simulink model "AnalysisSim"  (R2016a)
settings: Solver=VariableStepAuto  StartTime=0.0  StopTime=4.0  RelTol=1e-3
values from neighbouring files (symbols this model uses):
  C = Kphys    [DESIGN2_RobustFlutterSuppression-18-08-03.m]    (also in DESIGN2_RobustFlutterSuppression_18_08_03.m; Part1_Design_RobustFlutterSuppression.m; Part2_RobustnessAnalysis.m; ssctr.m = Ctmp)
  GeriFDsysPID2_IO = NdofwActSens(okeep,ikeep,AEC6,ModeShape,FEM,Vmps,aeroProp,massProp,     coeffdataPIDfull,actdata,sensdata)    [GenerateGeriModel.m]
  K = K*OutputBlend    [DESIGN1_RobustFlutterSuppression-18-07-27.m]    (also in DESIGN2_RobustFlutterSuppression-18-08-03.m; DESIGN2_RobustFlutterSuppression_18_08_03.m; Part1_Design_RobustFlutterSuppression.m)
  Vinf = VV    [DESIGN2_RobustFlutterSuppression-18-08-03.m]    (also in DESIGN2_RobustFlutterSuppression_18_08_03.m; Part1_Design_RobustFlutterSuppression.m; Part2_RobustnessAnalysis.m)
libraries: simulink_extras x4, dspsigattribs x4, cstblocks x1
settings Model: Creator=Julian  LastModifiedBy=Julian
settings GRTTargetCC: GeneratePreprocessorConditionals=Use local settings

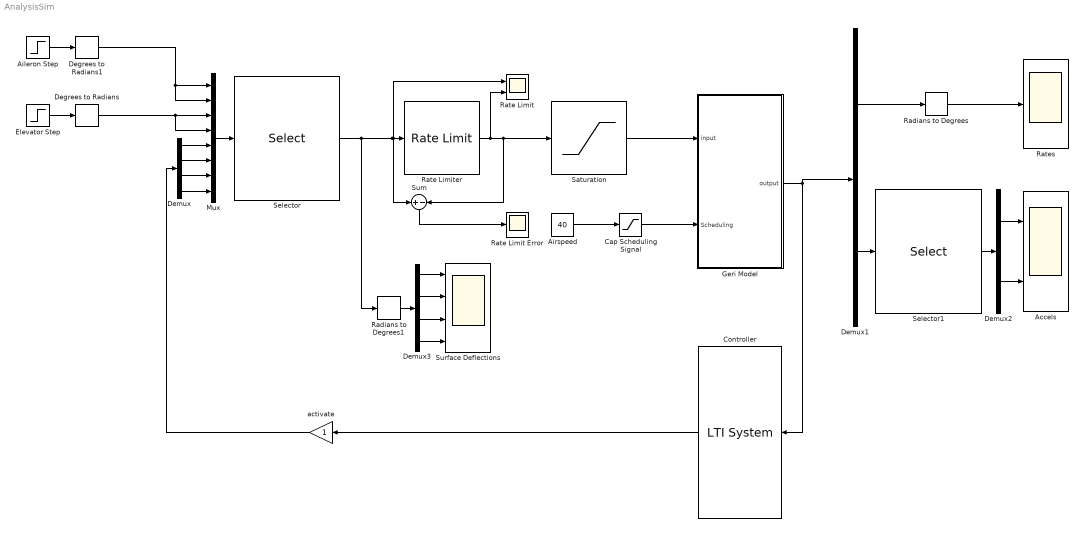
== system AnalysisSim ==
  Accels : Scope  NumInputPorts=2
  Aileron Step : Step  Time=3  After=0  SampleTime=0
  Airspeed : Constant  Value=40
  Cap Scheduling Signal : Saturate  UpperLimit=45  LowerLimit=25
  Controller : cstblocks/LTI System  sys=-C  IC=[]
  Degrees to Radians : simulink_extras/Transformations/Degrees to Radians
  Degrees to Radians1 : simulink_extras/Transformations/Degrees to Radians
  Demux : Demux
  Demux1 : Demux  Outputs=[2 6]
  Demux2 : Demux  Outputs=[3 3]
  Demux3 : Demux  Outputs=[2 2 2 2]
  Elevator Step : Step  SampleTime=0
  Geri Model : Subsystem
  Mux : Mux  Inputs=8
  Radians to Degrees : simulink_extras/Transformations/Radians to Degrees
  Radians to Degrees1 : simulink_extras/Transformations/Radians to Degrees
  Rate Limit : Scope  NumInputPorts=2
  Rate Limit Error : Scope
  Rate Limiter : RateLimiter  RisingSlewLimit=30/180*pi  FallingSlewLimit=-30/180*pi  SampleTimeMode=inherited
  Rates : Scope
  Saturation : Saturate  UpperLimit=30/180*pi  LowerLimit=-30/180*pi
  Selector : Selector  InputPortWidth=8  IndexOptions=Index vector (dialog)  Indices=[5 6 1 2 3 4 7 8]  OutputSizes=1
  Selector1 : Selector  InputPortWidth=6  IndexOptions=Index vector (dialog)  Indices=[6 2 5 4 1 3]  OutputSizes=1
  Sum : Sum  Inputs=+-
  Surface Deflections : Scope  NumInputPorts=4
  activate : Gain
  wires:
  Geri Model/1(output) -> Demux1/1, Controller/1
  Cap Scheduling Signal/1 -> Geri Model/2(Scheduling)
  Airspeed/1 -> Cap Scheduling Signal/1
  Mux/1 -> Selector/1
  Controller/1 -> activate/1
  Elevator Step/1 -> Degrees to Radians/1
  Demux/4 -> Mux/8
  Demux/3 -> Mux/7
  Demux/2 -> Mux/6
  Demux/1 -> Mux/5
  Degrees to Radians/1 -> Mux/4, Mux/3
  Aileron Step/1 -> Degrees to Radians1/1
  Degrees to Radians1/1 -> Mux/1, Mux/2
  Selector/1 -> Sum/1, Rate Limit/1, Rate Limiter/1, Radians to Degrees1/1
  Demux1/1 -> Radians to Degrees/1
  Demux1/2 -> Selector1/1
  Selector1/1 -> Demux2/1
  Demux2/1 -> Accels/1
  Demux2/2 -> Accels/2
  activate/1 -> Demux/1
  Radians to Degrees/1 -> Rates/1
  Radians to Degrees1/1 -> Demux3/1
  Demux3/1 -> Surface Deflections/1
  Demux3/3 -> Surface Deflections/3
  Demux3/2 -> Surface Deflections/2
  Demux3/4 -> Surface Deflections/4
  Saturation/1 -> Geri Model/1(input)
  Rate Limiter/1 -> Sum/2, Saturation/1, Rate Limit/2
  Sum/1 -> Rate Limit Error/1

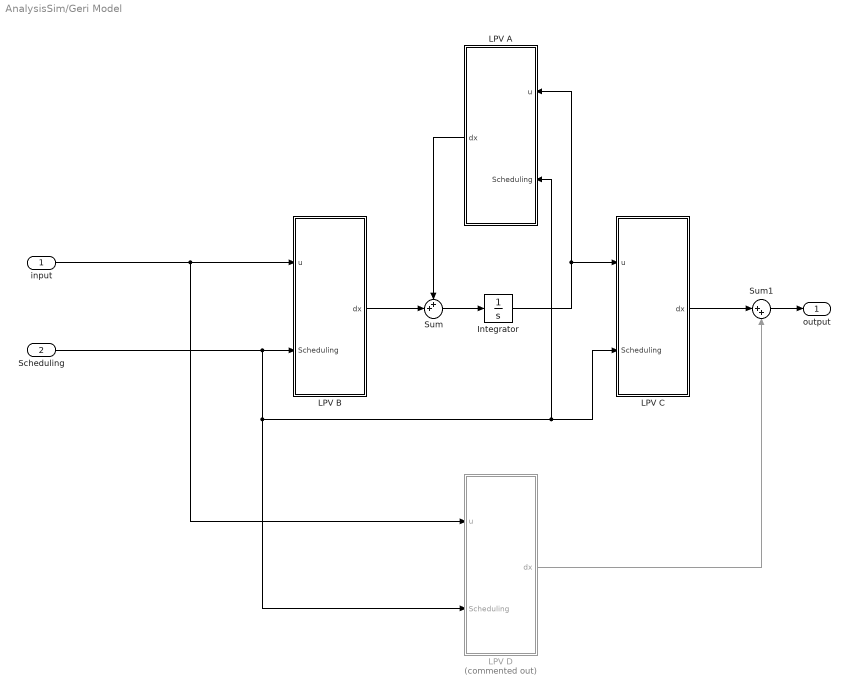
== system AnalysisSim/Geri Model ==
  input : Inport
  Scheduling : Inport  Port=2
  Integrator : Integrator  InitialCondition=zeros(size(GeriFDsysPID2_IO.a,1),1)
  LPV A : Subsystem
  LPV B : Subsystem
  LPV C : Subsystem
  LPV D : Subsystem  Commented=on
  Sum : Sum  Inputs=++|
  Sum1 : Sum  Inputs=|++
  output : Outport
  wires:
  LPV C/1(dx) -> Sum1/1
  Sum/1 -> Integrator/1
  Integrator/1 -> LPV C/1(u), LPV A/1(u)
  input/1 -> LPV D/1(u), LPV B/1(u)
  Scheduling/1 -> LPV B/2(Scheduling), LPV D/2(Scheduling), LPV C/2(Scheduling), LPV A/2(Scheduling)
  LPV B/1(dx) -> Sum/2
  LPV A/1(dx) -> Sum/1
  Sum1/1 -> output/1
  LPV D/1(dx) -> Sum1/2

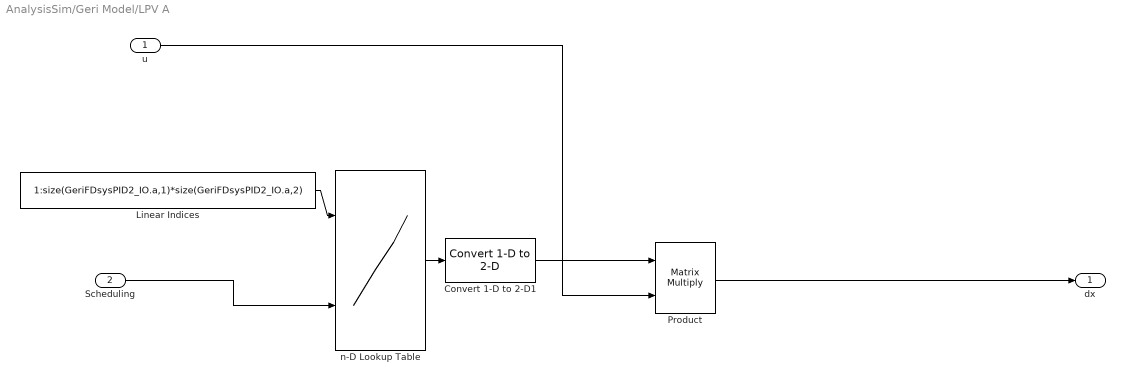
== system AnalysisSim/Geri Model/LPV A ==
  u : Inport
  Scheduling : Inport  Port=2
  Convert 1-D to 2-D1 : dspsigattribs/Convert 1-D to 2-D  M=size(GeriFDsysPID2_IO.a,1)  N=size(GeriFDsysPID2_IO.a,2)  frameBasedOut=off
  Linear Indices : Constant  Value=1:size(GeriFDsysPID2_IO.a,1)*size(GeriFDsysPID2_IO.a,2)
  Product : Product  Multiplication=Matrix(*)
  n-D Lookup Table : Lookup_n-D  BreakpointsForDimension1=1:size(GeriFDsysPID2_IO.a,1)*size(GeriFDsysPID2_IO.a,2)  BreakpointsForDimension2=Vinf  BreakpointsForDimension3=K.Parameter.q2.GridData  BreakpointsForDimension4=K.Parameter.q3.GridData  BreakpointsForDimension5=q3.GridData  BeginIndexSearchUsingPreviousIndexResult=on  Table=reshape(GeriFDsysPID2_IO.a,[size(GeriFDsysPID2_IO.a,1)*size(GeriFDsysPID2_IO.a,2), numel(Vinf)])  ExtrapMethod=Clip  UseLastTableValue=on  InternalRulePriority=Speed  RndMeth=Simplest  InputSameDT=on
  dx : Outport
  wires:
  Scheduling/1 -> n-D Lookup Table/2
  u/1 -> Product/2
  Linear Indices/1 -> n-D Lookup Table/1
  Convert 1-D to 2-D1/1 -> Product/1
  n-D Lookup Table/1 -> Convert 1-D to 2-D1/1
  Product/1 -> dx/1

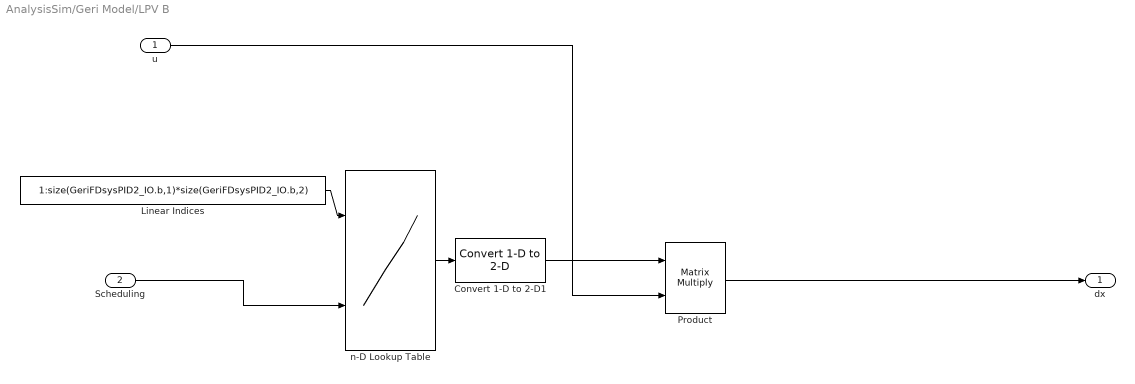
== system AnalysisSim/Geri Model/LPV B ==
  u : Inport
  Scheduling : Inport  Port=2
  Convert 1-D to 2-D1 : dspsigattribs/Convert 1-D to 2-D  M=size(GeriFDsysPID2_IO.b,1)  N=size(GeriFDsysPID2_IO.b,2)  frameBasedOut=off
  Linear Indices : Constant  Value=1:size(GeriFDsysPID2_IO.b,1)*size(GeriFDsysPID2_IO.b,2)
  Product : Product  Multiplication=Matrix(*)
  n-D Lookup Table : Lookup_n-D  BreakpointsForDimension1=1:size(GeriFDsysPID2_IO.b,1)*size(GeriFDsysPID2_IO.b,2)  BreakpointsForDimension2=Vinf  BreakpointsForDimension3=K.Parameter.q2.GridData  BreakpointsForDimension4=K.Parameter.q3.GridData  BreakpointsForDimension5=q3.GridData  BeginIndexSearchUsingPreviousIndexResult=on  Table=reshape(GeriFDsysPID2_IO.b,[size(GeriFDsysPID2_IO.b,1)*size(GeriFDsysPID2_IO.b,2), numel(Vinf)])  ExtrapMethod=Clip  UseLastTableValue=on  InternalRulePriority=Speed  RndMeth=Simplest  InputSameDT=on
  dx : Outport
  wires:
  Product/1 -> dx/1
  n-D Lookup Table/1 -> Convert 1-D to 2-D1/1
  Convert 1-D to 2-D1/1 -> Product/1
  Linear Indices/1 -> n-D Lookup Table/1
  u/1 -> Product/2
  Scheduling/1 -> n-D Lookup Table/2

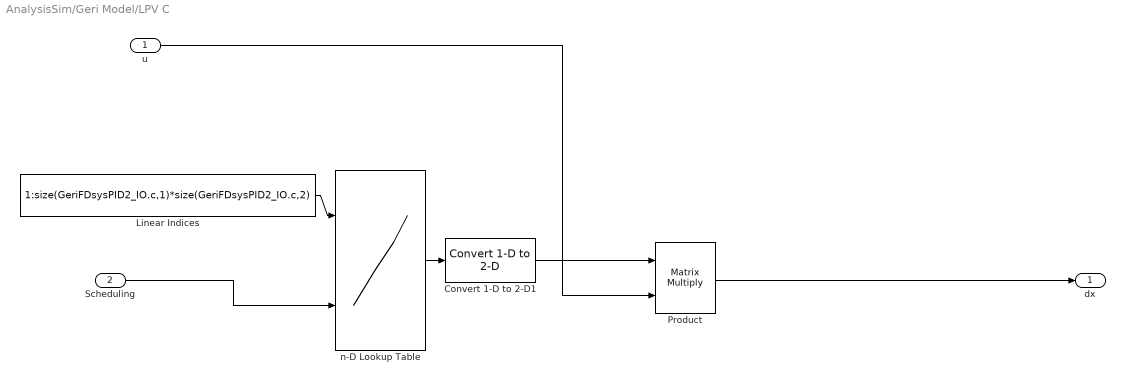
== system AnalysisSim/Geri Model/LPV C ==
  u : Inport
  Scheduling : Inport  Port=2
  Convert 1-D to 2-D1 : dspsigattribs/Convert 1-D to 2-D  M=size(GeriFDsysPID2_IO.c,1)  N=size(GeriFDsysPID2_IO.c,2)  frameBasedOut=off
  Linear Indices : Constant  Value=1:size(GeriFDsysPID2_IO.c,1)*size(GeriFDsysPID2_IO.c,2)
  Product : Product  Multiplication=Matrix(*)
  n-D Lookup Table : Lookup_n-D  BreakpointsForDimension1=1:size(GeriFDsysPID2_IO.c,1)*size(GeriFDsysPID2_IO.c,2)  BreakpointsForDimension2=Vinf  BreakpointsForDimension3=K.Parameter.q2.GridData  BreakpointsForDimension4=K.Parameter.q3.GridData  BreakpointsForDimension5=q3.GridData  Table=reshape(GeriFDsysPID2_IO.c,[size(GeriFDsysPID2_IO.c,1)*size(GeriFDsysPID2_IO.c,2), numel(Vinf)])  ExtrapMethod=Clip  UseLastTableValue=on  InternalRulePriority=Speed  RndMeth=Simplest  InputSameDT=on
  dx : Outport
  wires:
  Scheduling/1 -> n-D Lookup Table/2
  u/1 -> Product/2
  Linear Indices/1 -> n-D Lookup Table/1
  Convert 1-D to 2-D1/1 -> Product/1
  n-D Lookup Table/1 -> Convert 1-D to 2-D1/1
  Product/1 -> dx/1

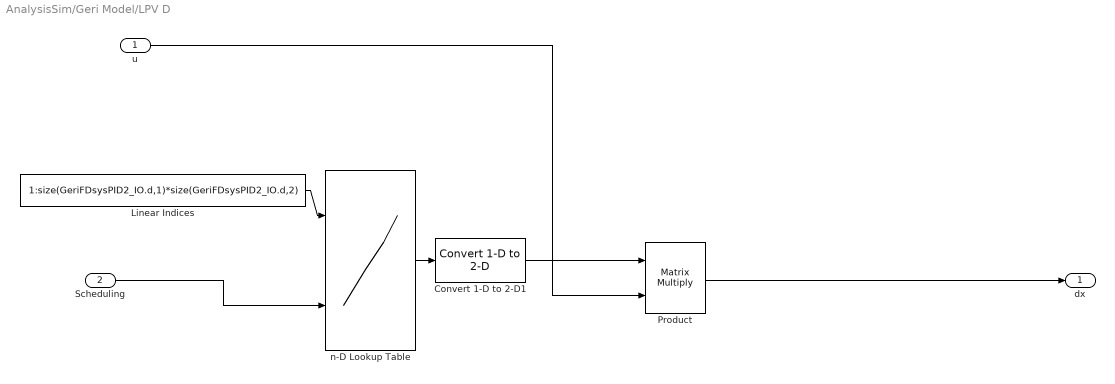
== system AnalysisSim/Geri Model/LPV D ==
  u : Inport
  Scheduling : Inport  Port=2
  Convert 1-D to 2-D1 : dspsigattribs/Convert 1-D to 2-D  M=size(GeriFDsysPID2_IO.d,1)  N=size(GeriFDsysPID2_IO.d,2)  frameBasedOut=off
  Linear Indices : Constant  Value=1:size(GeriFDsysPID2_IO.d,1)*size(GeriFDsysPID2_IO.d,2)
  Product : Product  Multiplication=Matrix(*)
  n-D Lookup Table : Lookup_n-D  BreakpointsForDimension1=1:size(GeriFDsysPID2_IO.d,1)*size(GeriFDsysPID2_IO.d,2)  BreakpointsForDimension2=Vinf  BreakpointsForDimension3=K.Parameter.q2.GridData  BreakpointsForDimension4=K.Parameter.q3.GridData  BreakpointsForDimension5=q3.GridData  Table=reshape(GeriFDsysPID2_IO.d,[size(GeriFDsysPID2_IO.d,1)*size(GeriFDsysPID2_IO.d,2), numel(Vinf)])  ExtrapMethod=Clip  UseLastTableValue=on  InternalRulePriority=Speed  RndMeth=Simplest  InputSameDT=on
  dx : Outport
  wires:
  Product/1 -> dx/1
  n-D Lookup Table/1 -> Convert 1-D to 2-D1/1
  Convert 1-D to 2-D1/1 -> Product/1
  Linear Indices/1 -> n-D Lookup Table/1
  u/1 -> Product/2
  Scheduling/1 -> n-D Lookup Table/2
